simulink model "standalone_battery_model"  (R2017a)
settings: Solver=ode4  StartTime=0.0  StopTime=end_time  FixedStep=sim_dt  RelTol=1e-3
undefined symbols (not defined in the file or in its folder): alpha_peukert, internal_resistance, max_cap_Ah, output_dt
libraries: dyn_lib x1
settings Model: Creator=Kevin  LastModifiedBy=Kevin
settings DataIOCC: ExternalInput=[throttle, airspeed_m_s, density_kg_m3]  LoadExternalInput=on  SignalLogging=off  DSMLogging=off

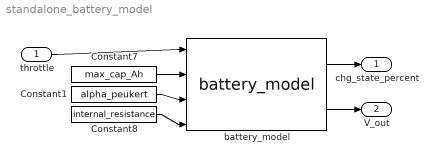
== system standalone_battery_model ==
  throttle : Inport
  Constant1 : Constant  Value=alpha_peukert
  Constant7 : Constant  Value=max_cap_Ah
  Constant8 : Constant  Value=internal_resistance
  battery_model : dyn_lib/battery_model
  chg_state_percent : Outport  SampleTime=output_dt
  V_out : Outport  Port=2  SampleTime=output_dt
  wires:
  throttle/1 -> battery_model/1
  battery_model/1 -> chg_state_percent/1
  battery_model/2 -> V_out/1
  Constant7/1 -> battery_model/2
  Constant1/1 -> battery_model/3
  Constant8/1 -> battery_model/4
